simulink model "Team_2_Strategy"  (Simulink 7.5)
settings: Solver=ode45  StartTime=0.0  StopTime=10.0  RelTol=1e-3
settings Model: Creator=smahapat  LastModifiedBy=pkodati
settings SolverCC: ZeroCrossControl=DisableAll
settings OptimizationCC: InlineParams=on

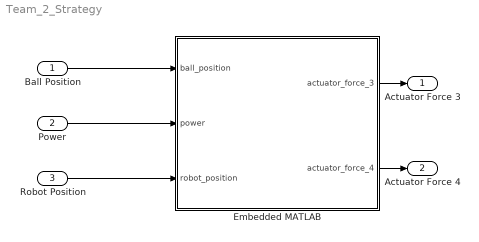
== system Team_2_Strategy ==
  Ball Position : Inport  PortDimensions=[2 1]
  Power : Inport  Port=2  UseBusObject=on  PortDimensions=[2 1]  BusOutputAsStruct=on
      settings: BusObject=Bus_Power
  Robot Position : Inport  Port=3  UseBusObject=on  PortDimensions=[4 1]
      settings: BusObject=Bus_Robot_Positions
  Embedded MATLAB : Stateflow chart  TreatAsAtomicUnit=on
  Actuator Force 3 : Outport
  Actuator Force 4 : Outport  Port=2
  wires:
  Embedded MATLAB/1(actuator_force_3) -> Actuator Force 3/1
  Power/1 -> Embedded MATLAB/2(power)
  Embedded MATLAB/2(actuator_force_4) -> Actuator Force 4/1
  Ball Position/1 -> Embedded MATLAB/1(ball_position)
  Robot Position/1 -> Embedded MATLAB/3(robot_position)

== matlab function Embedded MATLAB ==
  data: ball_position input double; power input double; robot_position input double; actuator_force_3 output double; actuator_force_4 output double
function [actuator_force_3, actuator_force_4] = fcn( ball_position,power, robot_position)
%#eml

d3=(robot_position(5:6,1)-ball_position);
d4=(robot_position(7:8,1)-ball_position);
if dot(d3,d3)>2
   actuator_force_3=-133*d3;
else
   r3=(ball_position- [0;50]);
   actuator_force_3=-65*r3;
end
if dot(d4,d4)>2
   actuator_force_4=-123*d4;
else
   r4=(ball_position- [0;50]);
   actuator_force_4=-25*r4;
end
